simulink model "Implementacion_Digital_OFDM"  (R2018b)
settings: Solver=ode5  StartTime=0.0  StopTime=N*Tb  FixedStep=Tsampling  RelTol=1e-3
values from neighbouring files (symbols this model uses):
  CantIFFT = 8    [Script_Implementacion_Digital.m]
  Eb = 4    [Script_Implementacion_Digital.m]
  Fp = Rb    (= 16000)    [Script_Implementacion_Digital.m]
  Tb = 1/Rb    (= 6.25e-05)    [Script_Implementacion_Digital.m]
libraries: commdigbbndpm3 x16, simulink x3, powerlib_meascontrol x2, dspxfrm3 x2, dspsigops x2, commrandsrc3 x1, commutil2 x1
settings Model: Creator=lukit  LastModifiedBy=lukit

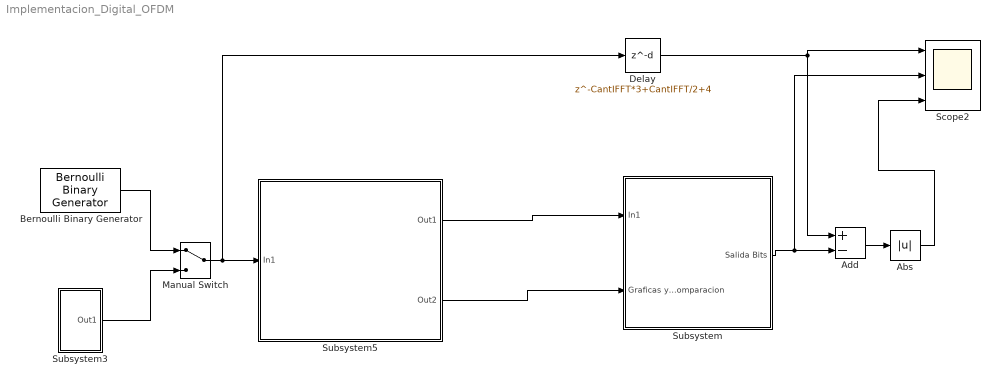
== system Implementacion_Digital_OFDM ==
  Abs : Abs
  Add : Sum  Inputs=+-
  Bernoulli Binary Generator : commrandsrc3/Bernoulli Binary Generator  ProbabilityOfZero=0.5  SeedSource=Auto  Seed=0  SampleTime=Tb  SamplesPerFrame=1  OutputDataType=double  SimulateUsing=Interpreted execution
      settings: SourceProductName=Communications Toolbox
  Delay : Delay  DelayLength=CantIFFT*3+CantIFFT/2+4  InitialCondition=0
  Manual Switch : ManualSwitch
  Scope2 : Scope  NumInputPorts=3
  Subsystem : Subsystem
  Subsystem3 : Subsystem
  Subsystem5 : Subsystem
  wires:
  Subsystem3/1(Out1) -> Manual Switch/2
  Manual Switch/1 -> Delay/1, Subsystem5/1(In1)
  Subsystem5/1(Out1) -> Subsystem/1(In1)
  Subsystem/1(Salida Bits) -> Scope2/2, Add/2
  Delay/1 -> Add/1, Scope2/1
  Add/1 -> Abs/1
  Abs/1 -> Scope2/3
  Subsystem5/2(Out2) -> Subsystem/2(Graficas y Comparacion)
  Bernoulli Binary Generator/1 -> Manual Switch/1

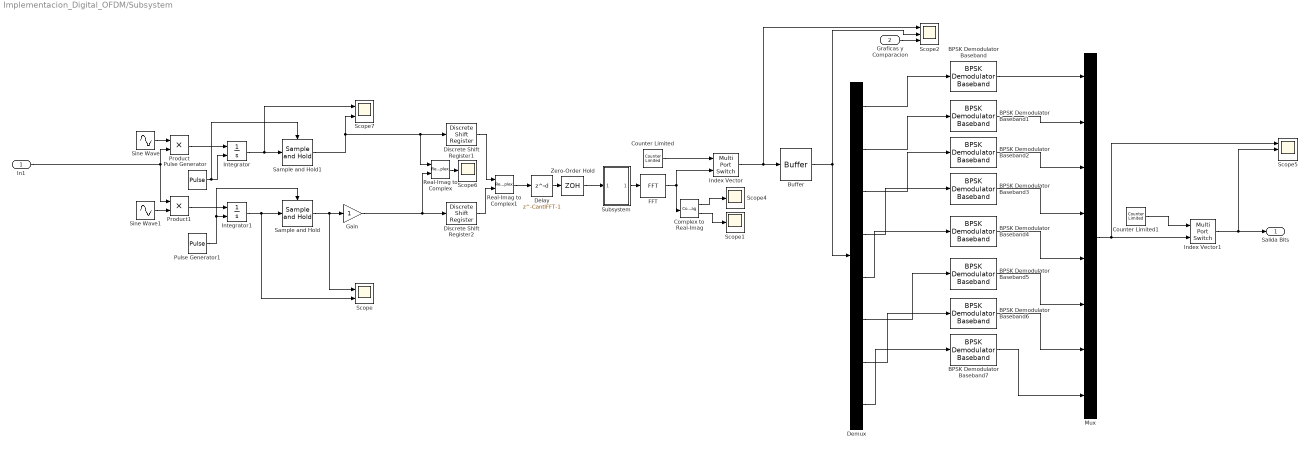
== system Implementacion_Digital_OFDM/Subsystem ==
  In1 : Inport
  Graficas y Comparacion : Inport  Port=2
  BPSK Demodulator Baseband{,1..7} (8 alike) : commdigbbndpm3/BPSK Demodulator Baseband  DecType=Hard decision  VarSource=Dialog  Variance=1  Ph=0  outDtype=Inherit via internal rule  derotateFactorWordLen=16  derotateFactorDataTypeStr=Inherit: Same word length as input  derotateFactorLastDataTypeStr=Inherit: Same word length as input
      settings: SourceProductName=Communications Toolbox
  Buffer : Buffer  N=CantIFFT  OutputFrames=off
  Complex to Real-Imag : ComplexToRealImag
  Counter Limited : simulink/Sources/Counter Limited  uplimit=CantIFFT-1  tsamp=Tb
  Counter Limited1 : simulink/Sources/Counter Limited  uplimit=CantIFFT-1  tsamp=Tb
  Delay : Delay  DelayLength=CantIFFT-1  InitialCondition=0
  Demux : Demux  Outputs=CantIFFT
  Discrete Shift Register1 : powerlib_meascontrol/Additional Components/Discrete Shift Register  NSamples=CantIFFT  InitialValue=0  Ts=Tb
      settings: SourceProductName=Simscape Electrical  SourceProductBaseCode=PS
  Discrete Shift Register2 : powerlib_meascontrol/Additional Components/Discrete Shift Register  NSamples=CantIFFT  InitialValue=0  Ts=Tb
      settings: SourceProductName=Simscape Electrical  SourceProductBaseCode=PS
  FFT : dspxfrm3/FFT  FFTImplementation=Auto  CompMethod=Table lookup  TableOpt=NEW  TableOptActive=Speed  BitRevOrder=off  Normalize=off  InheritFFTLength=off  FFTLength=CantIFFT  WrapInput=on  roundingMode=Floor  overflowMode=off  firstCoeffDataTypeStr=Inherit: Same word length as input  firstCoeffLastDataTypeStr=Inherit: Same word length as input  outputMin=[]  outputMax=[]
  Gain : Gain
  Index Vector : MultiPortSwitch  DataPortOrder=Zero-based contiguous  Inputs=1  zeroidx=on
  Index Vector1 : MultiPortSwitch  DataPortOrder=Zero-based contiguous  Inputs=1  zeroidx=on
  Integrator : Integrator  ExternalReset=rising
  Integrator1 : Integrator  ExternalReset=rising
  Mux : Mux  Inputs=CantIFFT
  Product : Product
  Product1 : Product
  Pulse Generator : DiscretePulseGenerator  PulseType=Time based  Period=Tb  PulseWidth=99.9
  Pulse Generator1 : DiscretePulseGenerator  PulseType=Time based  Period=Tb  PulseWidth=99.9
  Real-Imag to Complex : RealImagToComplex
  Real-Imag to Complex1 : RealImagToComplex
  Sample and Hold : dspsigops/Sample and Hold  trig=Falling edge  initCond=0  latchinput=off
  Sample and Hold1 : dspsigops/Sample and Hold  trig=Falling edge  initCond=0  latchinput=off
  Scope : Scope  NumInputPorts=2
  Scope1 : Scope
  Scope2 : Scope  NumInputPorts=3
  Scope4 : Scope
  Scope5 : Scope  NumInputPorts=3
  Scope6 : Scope
  Scope7 : Scope  NumInputPorts=2
  Sine Wave : Sin  Amplitude=sqrt(2/Tb)  Frequency=2*pi*(Fp)  Phase=pi/2
  Sine Wave1 : Sin  Amplitude=sqrt(2/Tb)  Frequency=2*pi*(Fp)
  Subsystem : Subsystem
  Zero-Order Hold : ZeroOrderHold  SampleTime=CantIFFT*Tb
  Salida Bits : Outport
  wires:
  Product/1 -> Integrator/1
  Sine Wave1/1 -> Product1/2
  Index Vector/1 -> Scope2/1, Buffer/1
  FFT/1 -> Complex to Real-Imag/1, Index Vector/2
  Discrete Shift Register1/1 -> Real-Imag to Complex1/1
  Counter Limited/1 -> Index Vector/1
  In1/1 -> Product1/1, Product/2
  Zero-Order Hold/1 -> Subsystem/1(In1)
  BPSK Demodulator Baseband1/1 -> Mux/2
  Mux/1 -> Scope5/1, Index Vector1/2
  Real-Imag to Complex/1 -> Scope6/1
  Sample and Hold/1 -> Scope/1, Gain/1
  BPSK Demodulator Baseband2/1 -> Mux/3
  Complex to Real-Imag/2 -> Scope1/1
  Integrator1/1 -> Scope/2, Sample and Hold/1
  Sine Wave/1 -> Product/1
  Pulse Generator1/1 -> Integrator1/2, Sample and Hold/Trigger
  BPSK Demodulator Baseband6/1 -> Mux/7
  Pulse Generator/1 -> Integrator/2, Sample and Hold1/Trigger
  Integrator/1 -> Scope7/1, Sample and Hold1/1
  Delay/1 -> Zero-Order Hold/1
  BPSK Demodulator Baseband5/1 -> Mux/6
  Real-Imag to Complex1/1 -> Delay/1
  Complex to Real-Imag/1 -> Scope4/1
  BPSK Demodulator Baseband7/1 -> Mux/8
  Product1/1 -> Integrator1/1
  Discrete Shift Register2/1 -> Real-Imag to Complex1/2
  Counter Limited1/1 -> Index Vector1/1
  BPSK Demodulator Baseband4/1 -> Mux/5
  Buffer/1 -> Scope2/2, Demux/1
  BPSK Demodulator Baseband3/1 -> Mux/4
  Index Vector1/1 -> Scope5/2, Salida Bits/1
  Sample and Hold1/1 -> Scope7/2, Real-Imag to Complex/1, Discrete Shift Register1/1
  Gain/1 -> Real-Imag to Complex/2, Discrete Shift Register2/1
  BPSK Demodulator Baseband/1 -> Mux/1
  Graficas y Comparacion/1 -> Scope2/3
  Subsystem/1(Out1) -> FFT/1
  Demux/1 -> BPSK Demodulator Baseband/1
  Demux/2 -> BPSK Demodulator Baseband1/1
  Demux/3 -> BPSK Demodulator Baseband2/1
  Demux/4 -> BPSK Demodulator Baseband3/1
  Demux/5 -> BPSK Demodulator Baseband4/1
  Demux/6 -> BPSK Demodulator Baseband5/1
  Demux/7 -> BPSK Demodulator Baseband6/1
  Demux/8 -> BPSK Demodulator Baseband7/1

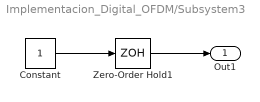
== system Implementacion_Digital_OFDM/Subsystem3 ==
  Constant : Constant  SampleTime=Tb
  Zero-Order Hold1 : ZeroOrderHold  SampleTime=-1
  Out1 : Outport
  wires:
  Constant/1 -> Zero-Order Hold1/1
  Zero-Order Hold1/1 -> Out1/1

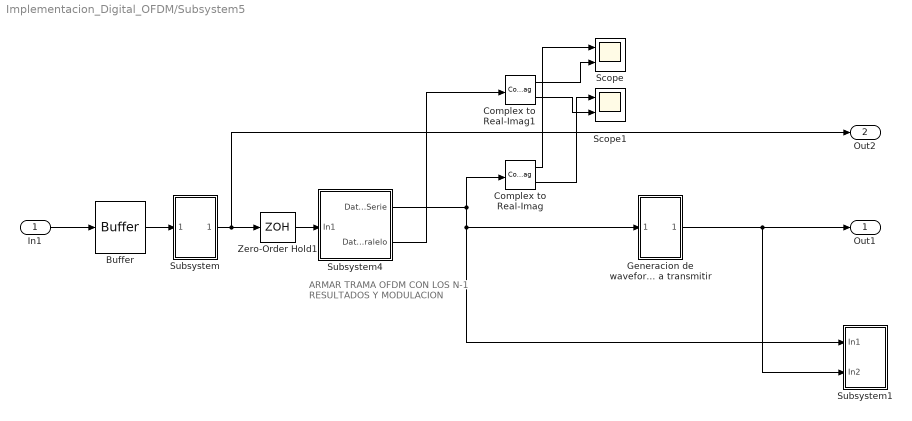
== system Implementacion_Digital_OFDM/Subsystem5 ==
  note: ARMAR TRAMA OFDM
      |  CON LOS N-1 RESULTADOS Y
      | MODULACION
  In1 : Inport
  Buffer : Buffer  N=CantIFFT  OutputFrames=off
  Complex to Real-Imag : ComplexToRealImag
  Complex to Real-Imag1 : ComplexToRealImag
  Generacion de waveform a transmitir : Subsystem
  Scope : Scope  NumInputPorts=2
  Scope1 : Scope  NumInputPorts=2
  Subsystem : Subsystem
  Subsystem1 : Subsystem
  Subsystem4 : Subsystem
  Zero-Order Hold1 : ZeroOrderHold  SampleTime=CantIFFT*Tb
  Out1 : Outport
  Out2 : Outport  Port=2
  wires:
  Buffer/1 -> Subsystem/1(In1)
  Generacion de waveform a transmitir/1(Out1) -> Subsystem1/2(In2), Out1/1
  Subsystem4/1(Datos Serie) -> Complex to Real-Imag/1, Subsystem1/1(In1), Generacion de waveform a transmitir/1(In1)
  In1/1 -> Buffer/1
  Subsystem/1(Out1) -> Out2/1, Zero-Order Hold1/1
  Zero-Order Hold1/1 -> Subsystem4/1(In1)
  Complex to Real-Imag/1 -> Scope/1
  Complex to Real-Imag/2 -> Scope1/1
  Complex to Real-Imag1/1 -> Scope/2
  Complex to Real-Imag1/2 -> Scope1/2
  Subsystem4/2(Datos paralelo) -> Complex to Real-Imag1/1

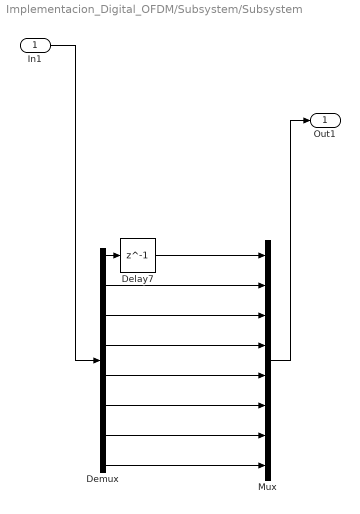
== system Implementacion_Digital_OFDM/Subsystem/Subsystem ==
  In1 : Inport
  Delay7 : Delay  DelayLength=1  InitialCondition=0
  Demux : Demux  Outputs=8
  Mux : Mux  Inputs=8
  Out1 : Outport
  wires:
  Delay7/1 -> Mux/1
  Demux/4 -> Mux/4
  Demux/2 -> Mux/2
  Demux/7 -> Mux/7
  Demux/1 -> Delay7/1
  Demux/5 -> Mux/5
  Demux/6 -> Mux/6
  Demux/3 -> Mux/3
  Demux/8 -> Mux/8
  In1/1 -> Demux/1
  Mux/1 -> Out1/1

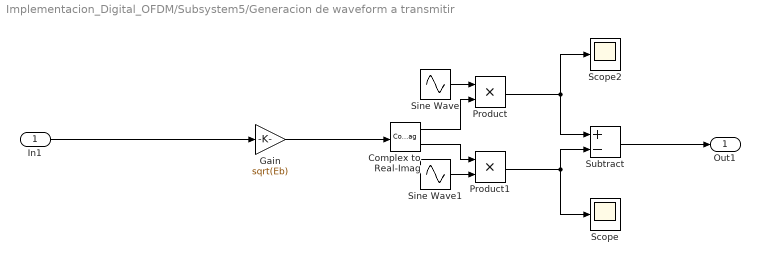
== system Implementacion_Digital_OFDM/Subsystem5/Generacion de waveform a transmitir ==
  In1 : Inport
  Complex to Real-Imag : ComplexToRealImag
  Gain : Gain  Gain=sqrt(Eb)
  Product : Product
  Product1 : Product
  Scope : Scope
  Scope2 : Scope
  Sine Wave : Sin  Amplitude=sqrt(2/Tb)  Frequency=2*pi*(Fp)  Phase=pi/2
  Sine Wave1 : Sin  Amplitude=sqrt(2/Tb)  Frequency=2*pi*(Fp)
  Subtract : Sum  Inputs=+-
  Out1 : Outport
  wires:
  Gain/1 -> Complex to Real-Imag/1
  Product/1 -> Subtract/1, Scope2/1
  Sine Wave1/1 -> Product1/2
  In1/1 -> Gain/1
  Sine Wave/1 -> Product/1
  Product1/1 -> Subtract/2, Scope/1
  Complex to Real-Imag/1 -> Product/2
  Subtract/1 -> Out1/1
  Complex to Real-Imag/2 -> Product1/1

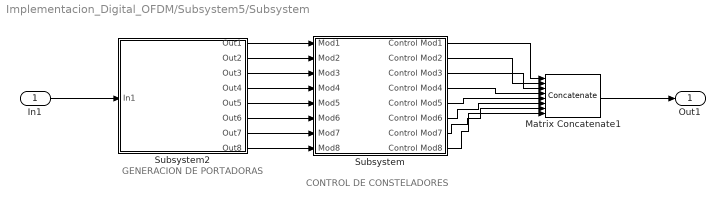
== system Implementacion_Digital_OFDM/Subsystem5/Subsystem ==
  note: CONTROL DE CONSTELADORES
  note: GENERACION DE PORTADORAS
  In1 : Inport
  Matrix Concatenate1 : Concatenate  NumInputs=CantIFFT
  Subsystem : Subsystem
  Subsystem2 : Subsystem
  Out1 : Outport
  wires:
  Subsystem/8(Control Mod8) -> Matrix Concatenate1/8
  Subsystem2/8(Out8) -> Subsystem/8(Mod8)
  In1/1 -> Subsystem2/1(In1)
  Subsystem/1(Control Mod1) -> Matrix Concatenate1/1
  Subsystem2/6(Out6) -> Subsystem/6(Mod6)
  Matrix Concatenate1/1 -> Out1/1
  Subsystem/6(Control Mod6) -> Matrix Concatenate1/6
  Subsystem/3(Control Mod3) -> Matrix Concatenate1/3
  Subsystem2/2(Out2) -> Subsystem/2(Mod2)
  Subsystem/2(Control Mod2) -> Matrix Concatenate1/2
  Subsystem2/3(Out3) -> Subsystem/3(Mod3)
  Subsystem2/1(Out1) -> Subsystem/1(Mod1)
  Subsystem/4(Control Mod4) -> Matrix Concatenate1/4
  Subsystem/5(Control Mod5) -> Matrix Concatenate1/5
  Subsystem2/4(Out4) -> Subsystem/4(Mod4)
  Subsystem2/7(Out7) -> Subsystem/7(Mod7)
  Subsystem2/5(Out5) -> Subsystem/5(Mod5)
  Subsystem/7(Control Mod7) -> Matrix Concatenate1/7

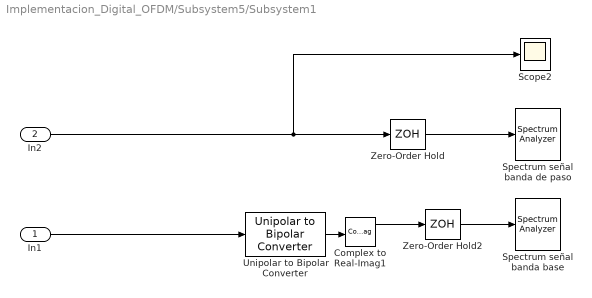
== system Implementacion_Digital_OFDM/Subsystem5/Subsystem1 ==
  In1 : Inport
  In2 : Inport  Port=2
  Complex to Real-Imag1 : ComplexToRealImag
  Scope2 : Scope
  Spectrum señal banda base : SpectrumAnalyzer
  Spectrum señal banda de paso : SpectrumAnalyzer
  Unipolar to Bipolar Converter : commutil2/Unipolar to Bipolar Converter  M=2  polarity=Positive  dataType=Inherit via internal rule
      settings: SourceProductName=Communications System Toolbox
  Zero-Order Hold : ZeroOrderHold  SampleTime=-1
  Zero-Order Hold2 : ZeroOrderHold  SampleTime=-1
  wires:
  Zero-Order Hold2/1 -> Spectrum señal banda base/1
  Unipolar to Bipolar Converter/1 -> Complex to Real-Imag1/1
  In2/1 -> Scope2/1, Zero-Order Hold/1
  Complex to Real-Imag1/1 -> Zero-Order Hold2/1
  Zero-Order Hold/1 -> Spectrum señal banda de paso/1
  In1/1 -> Unipolar to Bipolar Converter/1

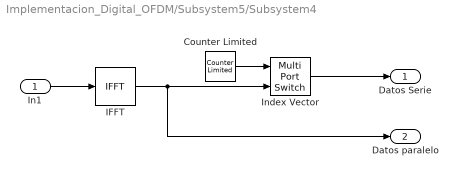
== system Implementacion_Digital_OFDM/Subsystem5/Subsystem4 ==
  In1 : Inport
  Counter Limited : simulink/Sources/Counter Limited  uplimit=CantIFFT-1  tsamp=Tb
  IFFT : dspxfrm3/IFFT  FFTImplementation=Auto  CompMethod=Table lookup  TableOpt=NEW  TableOptActive=Speed  BitRevOrder=off  cs_in=off  Normalize=on  InheritFFTLength=off  FFTLength=CantIFFT  WrapInput=on  mode=Complex  outSamplingMode=Sample based  roundingMode=Floor  overflowMode=off  firstCoeffDataTypeStr=Inherit: Same word length as input  firstCoeffLastDataTypeStr=Inherit: Same word length as input  outputMin=[]  outputMax=[]
      settings: SourceProductName=DSP System Toolbox
  Index Vector : MultiPortSwitch  DataPortOrder=Zero-based contiguous  Inputs=1  zeroidx=on
  Datos Serie : Outport
  Datos paralelo : Outport  Port=2
  wires:
  Counter Limited/1 -> Index Vector/1
  In1/1 -> IFFT/1
  Index Vector/1 -> Datos Serie/1
  IFFT/1 -> Datos paralelo/1, Index Vector/2

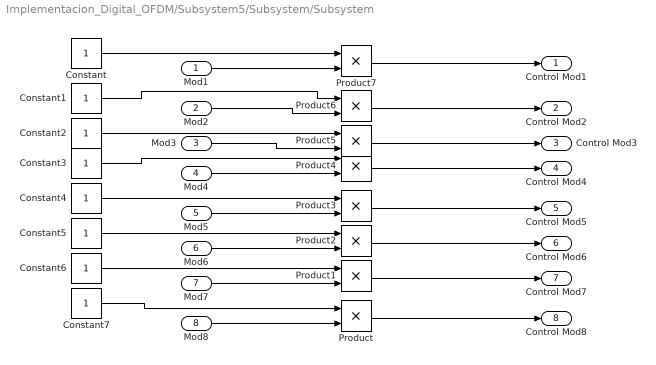
== system Implementacion_Digital_OFDM/Subsystem5/Subsystem/Subsystem ==
  Mod1 : Inport
  Mod2 : Inport  Port=2
  Mod3 : Inport  Port=3
  Mod4 : Inport  Port=4
  Mod5 : Inport  Port=5
  Mod6 : Inport  Port=6
  Mod7 : Inport  Port=7
  Mod8 : Inport  Port=8
  Constant{,1..7} (8 alike) : Constant  SampleTime=-1
  Product{,1..7} (8 alike) : Product
  Control Mod1 : Outport
  Control Mod2 : Outport  Port=2
  Control Mod3 : Outport  Port=3
  Control Mod4 : Outport  Port=4
  Control Mod5 : Outport  Port=5
  Control Mod6 : Outport  Port=6
  Control Mod7 : Outport  Port=7
  Control Mod8 : Outport  Port=8
  wires:
  Constant1/1 -> Product6/1
  Constant4/1 -> Product3/1
  Mod2/1 -> Product6/2
  Product7/1 -> Control Mod1/1
  Constant3/1 -> Product4/1
  Mod7/1 -> Product1/2
  Constant7/1 -> Product/1
  Mod5/1 -> Product3/2
  Mod6/1 -> Product2/2
  Mod8/1 -> Product/2
  Mod3/1 -> Product5/2
  Mod4/1 -> Product4/2
  Mod1/1 -> Product7/2
  Constant/1 -> Product7/1
  Constant6/1 -> Product1/1
  Constant5/1 -> Product2/1
  Constant2/1 -> Product5/1
  Product6/1 -> Control Mod2/1
  Product5/1 -> Control Mod3/1
  Product4/1 -> Control Mod4/1
  Product3/1 -> Control Mod5/1
  Product2/1 -> Control Mod6/1
  Product1/1 -> Control Mod7/1
  Product/1 -> Control Mod8/1

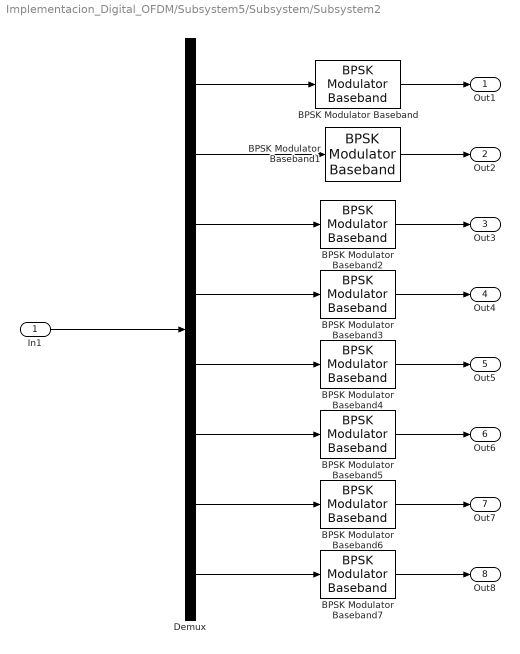
== system Implementacion_Digital_OFDM/Subsystem5/Subsystem/Subsystem2 ==
  In1 : Inport
  BPSK Modulator Baseband{,1..7} (8 alike) : commdigbbndpm3/BPSK Modulator Baseband  Ph=0  outDtype=double  outWordLen=16  outUDDataType=sfix(16)  outFracLenMode=Best precision  outFracLen=15  outDataTypeStr=double  outLastDataTypeStr=double
      settings: SourceProductName=Communications Toolbox
  Demux : Demux  Outputs=CantIFFT
  Out1 : Outport
  Out2 : Outport  Port=2
  Out3 : Outport  Port=3
  Out4 : Outport  Port=4
  Out5 : Outport  Port=5
  Out6 : Outport  Port=6
  Out7 : Outport  Port=7
  Out8 : Outport  Port=8
  wires:
  BPSK Modulator Baseband3/1 -> Out4/1
  BPSK Modulator Baseband7/1 -> Out8/1
  In1/1 -> Demux/1
  BPSK Modulator Baseband4/1 -> Out5/1
  BPSK Modulator Baseband6/1 -> Out7/1
  BPSK Modulator Baseband5/1 -> Out6/1
  BPSK Modulator Baseband1/1 -> Out2/1
  BPSK Modulator Baseband/1 -> Out1/1
  BPSK Modulator Baseband2/1 -> Out3/1
  Demux/1 -> BPSK Modulator Baseband/1
  Demux/2 -> BPSK Modulator Baseband1/1
  Demux/3 -> BPSK Modulator Baseband2/1
  Demux/4 -> BPSK Modulator Baseband3/1
  Demux/5 -> BPSK Modulator Baseband4/1
  Demux/6 -> BPSK Modulator Baseband5/1
  Demux/7 -> BPSK Modulator Baseband6/1
  Demux/8 -> BPSK Modulator Baseband7/1
